simulink model "Ulterasonic"  (R2021a)
settings: Solver=VariableStepAuto  StartTime=0.0  StopTime=10.0  RelTol=1e-3
values from neighbouring files (symbols this model uses):
  env = read_environment_data    [main.m]
  Selected_Env = 1    [main.m]
  Sensor_err = read_sensor_data    [main.m]
libraries: sharedtransform x1, dspsrcs4 x1
settings Model: Creator=mojta  LastModifiedBy=mojta

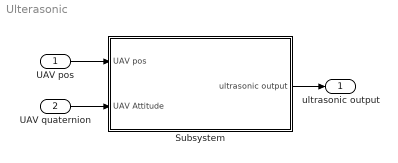
== system Ulterasonic ==
  UAV pos : Inport  PortDimensions=3
  UAV quaternion : Inport  Port=2  PortDimensions=4
  Subsystem : Subsystem
  ultrasonic output : Outport
  wires:
  UAV pos/1 -> Subsystem/1(UAV pos)
  Subsystem/1(ultrasonic output) -> ultrasonic output/1
  UAV quaternion/1 -> Subsystem/2(UAV Attitude)

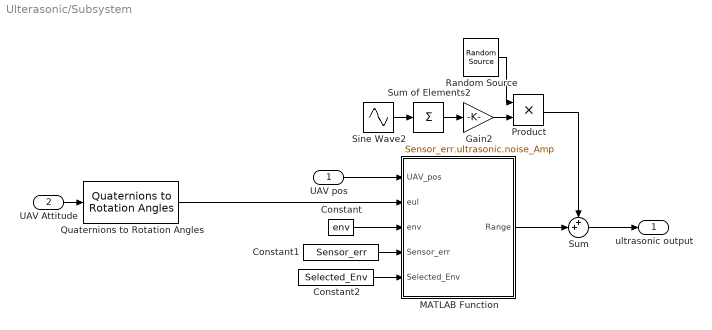
== system Ulterasonic/Subsystem ==
  UAV pos : Inport
  UAV Attitude : Inport  Port=2
  Constant : Constant  Value=env  VectorParams1D=off  OutDataTypeStr=Bus: env_bus
  Constant1 : Constant  Value=Sensor_err  VectorParams1D=off  OutDataTypeStr=Bus: Sensor_err_bus
  Constant2 : Constant  Value=Selected_Env
  Gain2 : Gain  Gain=Sensor_err.ultrasonic.noise_Amp
  MATLAB Function : MATLAB Function  TreatAsAtomicUnit=on
  Product : Product
  Quaternions to Rotation Angles : sharedtransform/Quaternions to Rotation Angles  rotationOrder=ZYX  aMode=aMode
      settings: SourceProductBaseCode=AE,PW,DR,MT,UV,VE
  Random Source : dspsrcs4/Random Source  SrcType=Uniform  NormMethod=Ziggurat  CltLength=12  MinVal=0  MaxVal=1  MeanVal=0  VarVal=1  RepMode=Not repeatable  rawSeed=1  IsInherit=off  SampMode=Discrete  SampTime=1  SampFrame=1  DataType=Double  OutComplex=Real  OutputFrames=off
  Sine Wave2 : Sin  Frequency=2*pi*Sensor_err.ultrasonic.freqs  SampleTime=0
  Sum : Sum  Inputs=++|
  Sum of Elements2 : Sum  Inputs=+
  ultrasonic output : Outport
  wires:
  Sum of Elements2/1 -> Gain2/1
  MATLAB Function/1(Range) -> Sum/2
  Sum/1 -> ultrasonic output/1
  Sine Wave2/1 -> Sum of Elements2/1
  Product/1 -> Sum/1
  Random Source/1 -> Product/1
  Gain2/1 -> Product/2
  UAV pos/1 -> MATLAB Function/1(UAV_pos)
  UAV Attitude/1 -> Quaternions to Rotation Angles/1
  Constant/1 -> MATLAB Function/3(env)
  Constant2/1 -> MATLAB Function/5(Selected_Env)
  Quaternions to Rotation Angles/1 -> MATLAB Function/2(eul)
  Constant1/1 -> MATLAB Function/4(Sensor_err)

== matlab function Ulterasonic/Subsystem/MATLAB Function ==
  settings: updateMethod=DISCRETE  sampleTime=0.1
  data: UAV_pos input; Range output size=1; eul input size=3; env input; Sensor_err input; Selected_Env input
function Range = ulteraSonicFcn(UAV_pos, eul, env, Sensor_err, Selected_Env)

% global Selected_Env Sensor_err  env

xu = UAV_pos(1);
yu = UAV_pos(2);
zu = UAV_pos(3);
psi   = eul(1);
theta = eul(2);

switch Selected_Env
    case 1
        if(norm(env.chimney1_1.pos - [xu yu]) < norm(env.chimney1_2.pos - [xu yu]))
            xc = env.chimney1_1.pos(1);
            yc = env.chimney1_1.pos(2);
            hc = env.chimney1_1.h;
            rc = env.chimney1_1.r;
        else
            xc = env.chimney1_2.pos(1);
            yc = env.chimney1_2.pos(2);
            hc = env.chimney1_2.h;
            rc = env.chimney1_2.r;
        end
    case 2
        if(norm(env.chimney2_1.pos - [xu yu]) < norm(env.chimney2_2.pos - [xu yu]))
            if(norm(env.chimney2_1.pos - [xu yu]) < norm(env.chimney2_3.pos - [xu yu]))
                xc = env.chimney2_1.pos(1);
                yc = env.chimney2_1.pos(2);
                hc = env.chimney2_1.h;
                rc = env.chimney2_1.r;
            else
                xc = env.chimney2_3.pos(1);
                yc = env.chimney2_3.pos(2);
                hc = env.chimney2_3.h;
                rc = env.chimney2_3.r;
            end
        else
            if(norm(env.chimney2_2.pos - [xu yu]) < norm(env.chimney2_3.pos - [xu yu]))
                xc = env.chimney2_2.pos(1);
                yc = env.chimney2_2.pos(2);
                hc = env.chimney2_2.h;
                rc = env.chimney2_2.r;
            else
                xc = env.chimney2_3.pos(1);
                yc = env.chimney2_3.pos(2);
                hc = env.chimney2_3.h;
                rc = env.chimney2_3.r;
            end
        end
    otherwise
        error("Wrong env has been Selected");
end

if(norm([xc-xu yc-yu])-rc > Sensor_err.ultrasonic.sup_range(2) || norm([xc-xu yc-yu])-rc < Sensor_err.ultrasonic.sup_range(1))
    Range = NaN;
else
    psi_rel  = abs(psi - atan2(yc-yu, xc-xu));
    xd       = norm([xc-xu yc-yu]);
    [xp, yp, psi_con_rel] = find_contact_point_on_circule(psi_rel, rc, xd);
    if ((psi_con_rel - abs(theta)) <65 *pi/180 || isnan(xp))
        Range = NaN;
    else
        zp = norm([xp yp])*tan(theta) + zu;
        Range = norm([xp yp zp]);
        if(Range > Sensor_err.ultrasonic.sup_range(2) || Range < Sensor_err.ultrasonic.sup_range(1) || zp > hc || rand > exp(-(90-psi_con_rel - abs(theta))).^2*0.005)
            Range = NaN;
        end
    end
end


end

function [xp, yp, psi_con_rel] = find_contact_point_on_circule(psi_rel, rc, xd)
a = abs(tan(psi_rel));

xp = min(roots([a^2+1 -2*xd xd^2-rc^2]));

if(imag(xp) ~= 0)
    xp = NaN;
    yp = NaN;
else
    yp = sqrt(rc^2 - (xd - xp)^2);
end

psi_con_rel = atan(-(0.5000*(2*xp - 2*xd))/(rc^2 - (xp - xd)^2)^0.5000) - psi_rel;

end
